simulink model "Deel2_volledig"  (R2020b)
settings: Solver=FixedStepAuto  StartTime=0.0  StopTime=10  FixedStep=0.001  RelTol=1e-3  EnableMultiTasking=on
libraries: fl_lib x10, nesl_utility x4
settings Model: Creator=Stino  LastModifiedBy=Stino
settings SolverCC: PositivePriorityOrder=on  AutoInsertRateTranBlk=on

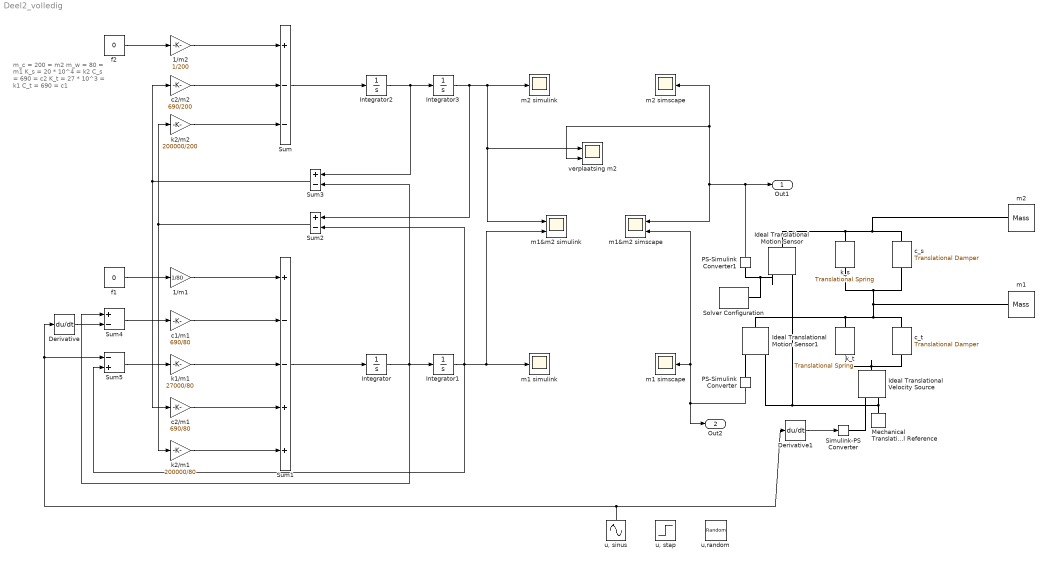
== system Deel2_volledig ==
  note: m_c = 200 = m2
      | m_w = 80 = m1
      | K_s = 20 * 10^4 = k2
      | C_s = 690 = c2
      | K_t = 27 * 10^3 = k1
      | C_t = 690 = c1
  1/m1 : Gain  Gain=1/80
  1/m2 : Gain  Gain=1/200
  Derivative : Derivative
  Derivative1 : Derivative
  Ideal Translational Motion Sensor : fl_lib/Mechanical/Mechanical Sensors/Ideal Translational Motion Sensor  offset=0 m
  Ideal Translational Motion Sensor1 : fl_lib/Mechanical/Mechanical Sensors/Ideal Translational Motion Sensor  offset=0 m
  Ideal Translational Velocity Source : fl_lib/Mechanical/Mechanical Sources/Ideal Translational Velocity Source
  Integrator{,1..3} (4 alike) : Integrator
  Mechanical Translational Reference : fl_lib/Mechanical/Translational Elements/Mechanical Translational Reference
  PS-Simulink Converter : nesl_utility/PS-Simulink Converter  PhysicalDomain=network_engine_domain  SubClassName=ps_output  LeftPortType=input  RightPortType=output  PseudoPeriodic=off  Frequencies=[]  Unit=inherit  AffineConversion=off
  PS-Simulink Converter1 : nesl_utility/PS-Simulink Converter  PhysicalDomain=network_engine_domain  SubClassName=ps_output  LeftPortType=input  RightPortType=output  PseudoPeriodic=off  Frequencies=[]  Unit=inherit  AffineConversion=off
  Simulink-PS Converter : nesl_utility/Simulink-PS Converter  PhysicalDomain=network_engine_domain  SubClassName=ps_input  LeftPortType=input  RightPortType=output  PseudoPeriodic=off  Frequencies=[]  NoiseDistribution=none  NoiseParameters=[]  Unit=1  AffineConversion=off  FilteringAndDerivatives=provide  SimscapeFilterOrder=1  InputFilterTimeConstant=0.001  UdotUserProvided=0
  Solver Configuration : nesl_utility/Solver Configuration  PhysicalDomain=network_engine_domain  SubClassName=solver  LeftPortType=input  RightPortType=generic  Tones=[]  Harmonics=[]  SimulateNoise=off  Profile=off  UseLocalSampling=off  EnableSwitchedLinearOptims=on  FrequencyDomain=off  UseCCode=off  RelTol=0.001  AbsTol=1e-06  MinStep=1e-09  ToWorkspace=off  RevertToSquareIcSolve=off  NumHomotopyIterations=100  PhasorMode=off  PhasorModeNumHarmonics=1  DoDC=off  ResidualTolerance=1e-09  UseLocalSolver=on  LocalSolverChoice=NE_BACKWARD_EULER_ADVANCER  LocalSolverSampleTime=0.001  DoFixedCost=on  MaxNonlinIter=3  MaxModeIter=2  ComputeImpulses=off  ImpulseIterations=2  LinearAlgebra=auto  EquationFormulation=NE_TIME_EF  DelaysMemoryBudget=1024  AutomaticFiltering=on  FilteringTimeConstant=0.001  PartitionStorageMethod=AS_NEEDED  PartitionMemoryBudget=1024  PartitionMethod=ROBUST
  Sum : Sum  Inputs=+--
  Sum1 : Sum  Inputs=+--++
  Sum2 : Sum  Inputs=+-
  Sum3 : Sum  Inputs=+-
  Sum4 : Sum  Inputs=+-
  Sum5 : Sum  Inputs=-+
  c1/m1 : Gain  Gain=690/80
  c2/m1 : Gain  Gain=690/80
  c2/m2 : Gain  Gain=690/200
  c_s : fl_lib/Mechanical/Translational Elements/Translational Damper  D=690 N/(m/s)  v_specify=off  v_priority=None  v=0 m/s  v_nominal_specify=off  v_nominal_unit=m/s  v_nominal_value=1  f_specify=off  f_priority=None  f=0 N  f_nominal_specify=off  f_nominal_unit=N  f_nominal_value=1
  c_t : fl_lib/Mechanical/Translational Elements/Translational Damper  D=690 N/(m/s)  v_specify=off  v_priority=None  v=0 m/s  v_nominal_specify=off  v_nominal_unit=m/s  v_nominal_value=1  f_specify=off  f_priority=None  f=0 N  f_nominal_specify=off  f_nominal_unit=N  f_nominal_value=1
  f1 : Constant  Value=0
  f2 : Constant  Value=0
  k1/m1 : Gain  Gain=27000/80
  k2/m1 : Gain  Gain=200000/80
  k2/m2 : Gain  Gain=200000/200
  k_s : fl_lib/Mechanical/Translational Elements/Translational Spring  spr_rate=200000 N/m  v_specify=off  v_priority=None  v=0 m/s  v_nominal_specify=off  v_nominal_unit=m/s  v_nominal_value=1  f_specify=off  f_priority=None  f=0 N  f_nominal_specify=off  f_nominal_unit=N  f_nominal_value=1  x_specify=off  x_priority=High  x=0 m  x_nominal_specify=off  x_nominal_unit=m  x_nominal_value=1
  k_t : fl_lib/Mechanical/Translational Elements/Translational Spring  spr_rate=27000 N/m  v_specify=off  v_priority=None  v=0 m/s  v_nominal_specify=off  v_nominal_unit=m/s  v_nominal_value=1  f_specify=off  f_priority=None  f=0 N  f_nominal_specify=off  f_nominal_unit=N  f_nominal_value=1  x_specify=off  x_priority=High  x=0 m  x_nominal_specify=off  x_nominal_unit=m  x_nominal_value=1
  m1 : fl_lib/Mechanical/Translational Elements/Mass  mass=80 kg  num_ports=foundation.enum.numPorts2.one  v_specify=off  v_priority=High  v=0 m/s  v_nominal_specify=off  v_nominal_unit=m/s  v_nominal_value=1  f_specify=off  f_priority=None  f=0 N  f_nominal_specify=off  f_nominal_unit=N  f_nominal_value=1
  m1 simscape : Scope
  m1 simulink : Scope
  m1&m2 simscape : Scope  NumInputPorts=2
  m1&m2 simulink : Scope  NumInputPorts=2
  m2 : fl_lib/Mechanical/Translational Elements/Mass  mass=200 kg  num_ports=foundation.enum.numPorts2.one  v_specify=off  v_priority=High  v=0 m/s  v_nominal_specify=off  v_nominal_unit=m/s  v_nominal_value=1  f_specify=off  f_priority=None  f=0 N  f_nominal_specify=off  f_nominal_unit=N  f_nominal_value=1
  m2 simscape : Scope
  m2 simulink : Scope
  "u, sinus" : Sin  Amplitude=0.02  Frequency=31.416  SampleTime=0
  "u, stap" : Step  Time=5  After=0.05  SampleTime=0
  u,random : UniformRandomNumber  Minimum=0  Maximum=0.02  SampleTime=0.1
  verplaatsing m2 : Scope  NumInputPorts=2
  Out1 : Outport
  Out2 : Outport  Port=2
  wires:
  k2/m2/1 -> Sum/3
  c2/m2/1 -> Sum/2
  1/m2/1 -> Sum/1
  k2/m1/1 -> Sum1/5
  c2/m1/1 -> Sum1/4
  k1/m1/1 -> Sum1/3
  c1/m1/1 -> Sum1/2
  1/m1/1 -> Sum1/1
  f2/1 -> 1/m2/1
  Sum1/1 -> Integrator/1
  Integrator/1 -> Sum3/2, Sum4/1, Integrator1/1
  Sum/1 -> Integrator2/1
  Integrator2/1 -> Sum3/1, Integrator3/1
  Integrator3/1 -> Sum2/1, m1&m2 simulink/1, verplaatsing m2/1, m2 simulink/1
  f1/1 -> 1/m1/1
  Sum4/1 -> c1/m1/1
  Sum5/1 -> k1/m1/1
  Sum3/1 -> c2/m1/1, c2/m2/1
  Sum2/1 -> k2/m1/1, k2/m2/1
  Derivative/1 -> Sum4/2
  "u, sinus"/1 -> Derivative1/1, Derivative/1, Sum5/1
  Derivative1/1 -> Simulink-PS Converter/1
  PS-Simulink Converter/1 -> m1&m2 simscape/2, m1 simscape/1, Out2/1
  PS-Simulink Converter1/1 -> verplaatsing m2/2, m2 simscape/1, m1&m2 simscape/1, Out1/1
  Integrator1/1 -> Sum2/2, Sum5/2, m1&m2 simulink/2, m1 simulink/1
  connections:
  Simulink-PS Converter/RConn1 -- Ideal Translational Velocity Source/RConn1
  Ideal Translational Velocity Source/LConn1 -- k_t/RConn1 -- c_t/RConn1
  c_t/LConn1 -- Ideal Translational Motion Sensor1/LConn1 -- k_t/LConn1 -- m1/LConn1 -- k_s/RConn1 -- c_s/RConn1
  c_s/LConn1 -- m2/LConn1 -- Ideal Translational Motion Sensor/LConn1 -- k_s/LConn1
  Ideal Translational Velocity Source/RConn2 -- Ideal Translational Motion Sensor/RConn1 -- Ideal Translational Motion Sensor1/RConn1 -- Mechanical Translational Reference/LConn1
  PS-Simulink Converter/LConn1 -- Ideal Translational Motion Sensor1/RConn3
  Ideal Translational Motion Sensor/RConn3 -- Solver Configuration/RConn1 -- PS-Simulink Converter1/LConn1
